simulink model "SSTI_DCDC_IET"  (R2021a)
settings: Solver=ode1  StartTime=0.0  StopTime=1.5  FixedStep=5e-6  RelTol=1e-3
values from neighbouring files (symbols this model uses):
  Pn = 1000e6    (= 1000000000)    [main_DroopCtrl_inzFDPI.m]    (also in main_PU.m)
  Sr = 10e9    (= 10000000000)    [main.m]    (also in main_DroopCtrl_inzFDPI.m)
  SYS =     [Small signal model.mat]
  Vdc1_ref = 640e3    (= 640000)    [main_DroopCtrl_inzFDPI.m]    (also in main_PU.m)
  Vdc2_ref = 500e3    (= 500000)    [main_DroopCtrl_inzFDPI.m]    (also in main_PU.m)
settings Model: Creator=Util-SHAFIQUE  LastModifiedBy=Frederic_Colas
settings SolverCC: AlgebraicLoopSolver=TrustRegion

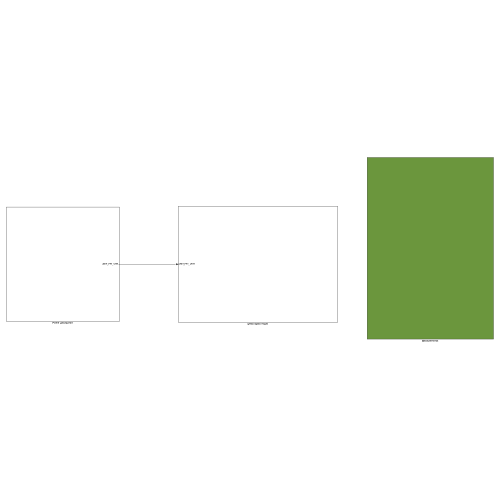
[thumbnail: Simulink's stored preview of the top-level diagram]
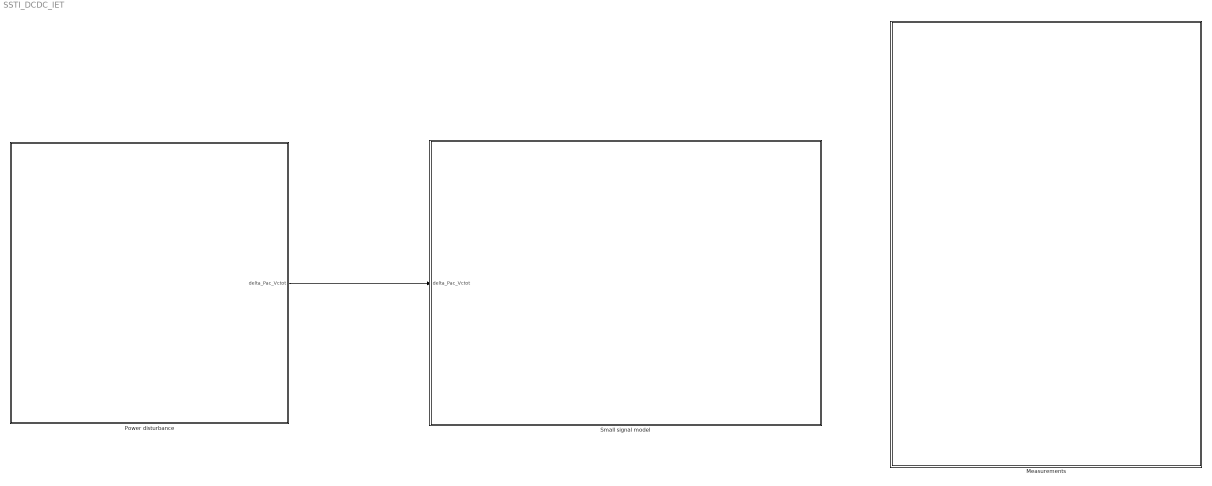
== system SSTI_DCDC_IET ==
  Measurements : Subsystem
  Power disturbance : Subsystem
  Small signal model : Subsystem
  wires:
  Power disturbance/1(delta_Pac_Vctot) -> Small signal model/1(delta_Pac_Vctot)

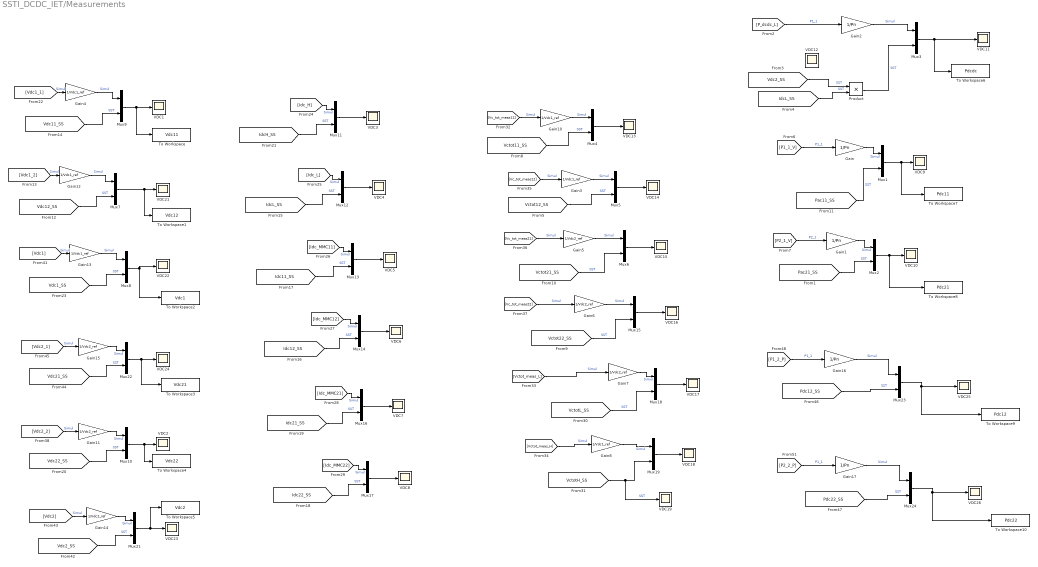
== system SSTI_DCDC_IET/Measurements ==
  Gain{,1..2,16..17} (5 alike) : Gain  Gain=1/Pn
  Gain{3..4,8,10,12..13} (6 alike) : Gain  Gain=1/Vdc1_ref
  Gain{5..7,11,14..15} (6 alike) : Gain  Gain=1/Vdc2_ref
  Mux{1..19,21..24} (23 alike) : Mux  Inputs=2
  Product : Product
  To Workspace : ToWorkspace  VariableName=Vdc11  SaveFormat=Structure With Time  SampleTime=-1
  To Workspace1 : ToWorkspace  VariableName=Vdc12  SaveFormat=Structure With Time  SampleTime=-1
  To Workspace10 : ToWorkspace  VariableName=Pdc22  SaveFormat=Structure With Time  SampleTime=-1
  To Workspace2 : ToWorkspace  VariableName=Vdc1  SaveFormat=Structure With Time  SampleTime=-1
  To Workspace3 : ToWorkspace  VariableName=Vdc21  SaveFormat=Structure With Time  SampleTime=-1
  To Workspace4 : ToWorkspace  VariableName=Vdc22  SaveFormat=Structure With Time  SampleTime=-1
  To Workspace5 : ToWorkspace  VariableName=Vdc2  SaveFormat=Structure With Time  SampleTime=-1
  To Workspace6 : ToWorkspace  VariableName=Pdcdc  SaveFormat=Structure With Time  SampleTime=-1
  To Workspace7 : ToWorkspace  VariableName=Pdc11  SaveFormat=Structure With Time  SampleTime=-1
  To Workspace8 : ToWorkspace  VariableName=Pdc21  SaveFormat=Structure With Time  SampleTime=-1
  To Workspace9 : ToWorkspace  VariableName=Pdc12  SaveFormat=Structure With Time  SampleTime=-1
  VDC{1..19,21..26} (25 alike) : Scope
  wires:
  Mux11/1 -> VDC3/1
  [Idc_L] -> Mux12/1  "Simul"
  Mux10/1 -> To Workspace4/1, VDC2/1
  [Idc_MMC12] -> Mux14/1  "Simul"
  [Vdc2_2] -> Gain11/1  "Simul"
  [Idc22_SS] -> Mux17/2  "SST"
  Mux17/1 -> VDC8/1
  Gain4/1 -> Mux9/1  "Simul"
  [Vc_tot_meas12] -> Gain3/1  "Simul"
  [Vdc1_1] -> Gain4/1  "Simul"
  Gain10/1 -> Mux4/1  "Simul"
  [Idc_H] -> Mux11/1  "Simul"
  [Vc_tot_meas21] -> Gain5/1  "Simul"
  [Vc_tot_meas11] -> Gain10/1  "Simul"
  [VctotH_SS] -> VDC19/1, Mux19/2  "SST"
  Gain3/1 -> Mux5/1  "Simul"
  Mux4/1 -> VDC13/1
  [Idc11_SS] -> Mux13/2  "SST"
  Mux12/1 -> VDC4/1
  [Idc21_SS] -> Mux16/2  "SST"
  Mux16/1 -> VDC7/1
  Mux6/1 -> VDC15/1
  Gain6/1 -> Mux15/1  "Simul"
  [Vctot22_SS] -> Mux15/2  "SST"
  Mux18/1 -> VDC17/1
  [Vctot12_SS] -> Mux5/2  "SST"
  [Vdc11_SS] -> Mux9/2  "SST"
  [IdcH_SS] -> Mux11/2  "SST"
  [Vctot11_SS] -> Mux4/2  "SST"
  Mux19/1 -> VDC18/1
  Gain5/1 -> Mux6/1  "Simul"
  [VctotL_SS] -> Mux18/2  "SST"
  Mux9/1 -> To Workspace/1, VDC1/1
  [Idc_MMC21] -> Mux16/1  "Simul"
  Gain7/1 -> Mux18/1  "Simul"
  Gain8/1 -> Mux19/1  "Simul"
  [Vctot21_SS] -> Mux6/2  "SST"
  [IdcL_SS] -> Mux12/2  "SST"
  Mux5/1 -> VDC14/1
  [Vctot_meas_L] -> Gain7/1  "Simul"
  Mux15/1 -> VDC16/1
  [Vctot_meas_H] -> Gain8/1  "Simul"
  [Vc_tot_meas22] -> Gain6/1  "Simul"
  Mux13/1 -> VDC5/1
  [Idc12_SS] -> Mux14/2  "SST"
  [Idc_MMC11] -> Mux13/1  "Simul"
  [Vdc22_SS] -> Mux10/2  "SST"
  Mux14/1 -> VDC6/1
  [Idc_MMC22] -> Mux17/1  "Simul"
  Gain11/1 -> Mux10/1  "Simul"
  [P2_1_V] -> Gain1/1  "P2_1"
  [Vdc2_SS] -> Product/1  "SST"
  Gain/1 -> Mux1/1  "Simul"
  [IdcL_SS] -> Product/2  "SST"
  [P1_1_V] -> Gain/1  "P1_1"
  Gain2/1 -> Mux3/1  "Simul"
  [Pac21_SS] -> Mux2/2  "SST"
  [Pac11_SS] -> Mux1/2  "SST"
  Gain1/1 -> Mux2/1  "Simul"
  Mux1/1 -> To Workspace7/1, VDC9/1
  Product/1 -> Mux3/2  "SST"
  [P_dcdc_L] -> Gain2/1  "P1_1"
  Mux2/1 -> To Workspace8/1, VDC10/1
  Mux3/1 -> To Workspace6/1, VDC11/1
  Mux7/1 -> To Workspace1/1, VDC21/1
  [Vdc12_SS] -> Mux7/2  "SST"
  [Vdc1_2] -> Gain12/1  "Simul"
  Gain12/1 -> Mux7/1  "Simul"
  Gain13/1 -> Mux8/1  "Simul"
  [Vdc1] -> Gain13/1  "Simul"
  [Vdc1_SS] -> Mux8/2  "SST"
  Mux8/1 -> To Workspace2/1, VDC22/1
  Gain14/1 -> Mux21/1  "Simul"
  [Vdc2_SS] -> Mux21/2  "SST"
  [Vdc2] -> Gain14/1  "Simul"
  Mux21/1 -> To Workspace5/1, VDC23/1
  Mux22/1 -> To Workspace3/1, VDC24/1
  [Vdc2_1] -> Gain15/1  "Simul"
  [Vdc21_SS] -> Mux22/2  "SST"
  Gain15/1 -> Mux22/1  "Simul"
  [P1_2_P] -> Gain16/1  "P1_1"
  Gain16/1 -> Mux23/1  "Simul"
  Mux23/1 -> To Workspace9/1, VDC25/1
  Mux24/1 -> VDC26/1, To Workspace10/1
  Gain17/1 -> Mux24/1  "Simul"
  [P2_2_P] -> Gain17/1  "P1_1"
  [Pdc12_SS] -> Mux23/2  "SST"
  [Pdc22_SS] -> Mux24/2  "SST"

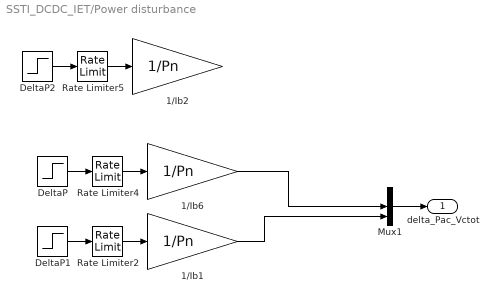
== system SSTI_DCDC_IET/Power disturbance ==
  1/Ib1 : Gain  Gain=1/Pn
  1/Ib2 : Gain  Gain=1/Pn
  1/Ib6 : Gain  Gain=1/Pn
  DeltaP : Step  Time=0.3  After=-50e6  SampleTime=0
  DeltaP1 : Step  After=50e6  SampleTime=0
  DeltaP2 : Step  Time=0.5  After=25e6  SampleTime=0
  Mux1 : Mux  Inputs=3
  Rate Limiter2 : RateLimiter  RisingSlewLimit=Sr  FallingSlewLimit=-Sr  SampleTimeMode=inherited
  Rate Limiter4 : RateLimiter  RisingSlewLimit=Sr  FallingSlewLimit=-Sr  SampleTimeMode=inherited
  Rate Limiter5 : RateLimiter  RisingSlewLimit=Sr  FallingSlewLimit=-Sr  SampleTimeMode=inherited
  delta_Pac_Vctot : Outport
  wires:
  DeltaP/1 -> Rate Limiter4/1
  DeltaP1/1 -> Rate Limiter2/1
  DeltaP2/1 -> Rate Limiter5/1
  1/Ib1/1 -> Mux1/3
  1/Ib6/1 -> Mux1/2
  Rate Limiter5/1 -> 1/Ib2/1
  Rate Limiter4/1 -> 1/Ib6/1
  Rate Limiter2/1 -> 1/Ib1/1
  Mux1/1 -> delta_Pac_Vctot/1

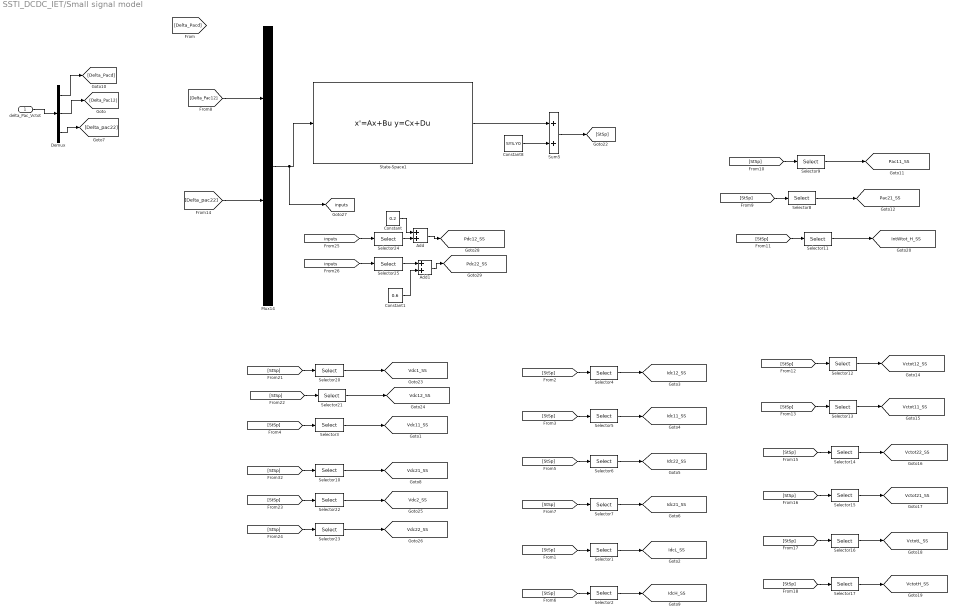
== system SSTI_DCDC_IET/Small signal model ==
  delta_Pac_Vctot : Inport
  Add : Sum
  Add1 : Sum
  Constant : Constant  Value=0.2
  Constant1 : Constant  Value=0.6
  Constant8 : Constant  Value=SYS.Y0
  Demux : Demux  Outputs=3
  Mux14 : Mux  Inputs=23
  Selector1 : Selector  InputPortWidth=46  IndexOptions=Index vector (dialog)  Indices=4  OutputSizes=1
  Selector10 : Selector  InputPortWidth=46  IndexOptions=Index vector (dialog)  Indices=43  OutputSizes=1
  Selector11 : Selector  InputPortWidth=46  IndexOptions=Index vector (dialog)  Indices=2  OutputSizes=1
  Selector12 : Selector  InputPortWidth=46  IndexOptions=Index vector (dialog)  Indices=12  OutputSizes=1
  Selector13 : Selector  InputPortWidth=46  IndexOptions=Index vector (dialog)  Indices=20  OutputSizes=1
  Selector14 : Selector  InputPortWidth=46  IndexOptions=Index vector (dialog)  Indices=32  OutputSizes=1
  Selector15 : Selector  InputPortWidth=46  IndexOptions=Index vector (dialog)  Indices=40  OutputSizes=1
  Selector16 : Selector  InputPortWidth=46  IndexOptions=Index vector (dialog)  Indices=3  OutputSizes=1
  Selector17 : Selector  InputPortWidth=46  IndexOptions=Index vector (dialog)  Indices=5  OutputSizes=1
  Selector2 : Selector  InputPortWidth=46  IndexOptions=Index vector (dialog)  Indices=6  OutputSizes=1
  Selector20 : Selector  InputPortWidth=46  IndexOptions=Index vector (dialog)  Indices=25  OutputSizes=1
  Selector21 : Selector  InputPortWidth=46  IndexOptions=Index vector (dialog)  Indices=24  OutputSizes=1
  Selector22 : Selector  InputPortWidth=46  IndexOptions=Index vector (dialog)  Indices=45  OutputSizes=1
  Selector23 : Selector  InputPortWidth=46  IndexOptions=Index vector (dialog)  Indices=44  OutputSizes=1
  Selector24 : Selector  InputPortWidth=23  IndexOptions=Index vector (dialog)  Indices=6  OutputSizes=1
  Selector25 : Selector  InputPortWidth=23  IndexOptions=Index vector (dialog)  Indices=15  OutputSizes=1
  Selector3 : Selector  InputPortWidth=46  IndexOptions=Index vector (dialog)  Indices=23  OutputSizes=1
  Selector4 : Selector  InputPortWidth=46  IndexOptions=Index vector (dialog)  Indices=14  OutputSizes=1
  Selector5 : Selector  InputPortWidth=46  IndexOptions=Index vector (dialog)  Indices=22  OutputSizes=1
  Selector6 : Selector  InputPortWidth=46  IndexOptions=Index vector (dialog)  Indices=34  OutputSizes=1
  Selector7 : Selector  InputPortWidth=46  IndexOptions=Index vector (dialog)  Indices=42  OutputSizes=1
  Selector8 : Selector  InputPortWidth=46  IndexOptions=Index vector (dialog)  Indices=46  OutputSizes=1
  Selector9 : Selector  InputPortWidth=46  IndexOptions=Index vector (dialog)  Indices=26  OutputSizes=1
  State-Space1 : StateSpace  A=SYS.A_sys  B=SYS.B_sys  C=SYS.C_sys  D=SYS.D_sys  InitialCondition=zeros(1,length(SYS.States.StrCell))
  Sum5 : Sum
  tag scope: Idc11_SS=global, Idc12_SS=global, Idc21_SS=global, Idc22_SS=global, IdcH_SS=global, IdcL_SS=global, IntWtot_H_SS=global, Pac11_SS=global, Pac21_SS=global, Pdc12_SS=global, Pdc22_SS=global, Vctot11_SS=global, Vctot12_SS=global, Vctot21_SS=global, Vctot22_SS=global, VctotH_SS=global, VctotL_SS=global, Vdc11_SS=global, Vdc12_SS=global, Vdc1_SS=global, Vdc21_SS=global, Vdc22_SS=global, Vdc2_SS=global, inputs=global
  wires:
  [StSp] -> Selector1/1
  Constant8/1 -> Sum5/2
  Selector1/1 -> [IdcL_SS]
  [StSp] -> Selector10/1
  State-Space1/1 -> Sum5/1
  Selector2/1 -> [IdcH_SS]
  Selector10/1 -> [Vdc21_SS]
  Mux14/1 -> [inputs], State-Space1/1
  Sum5/1 -> [StSp]
  [StSp] -> Selector2/1
  Selector3/1 -> [Vdc11_SS]
  [StSp] -> Selector3/1
  Demux/3 -> [Delta_pac22]
  Demux/2 -> [Delta_Pac12]
  [StSp] -> Selector5/1
  Selector5/1 -> [Idc11_SS]
  Selector4/1 -> [Idc12_SS]
  [StSp] -> Selector4/1
  [StSp] -> Selector6/1
  Selector6/1 -> [Idc22_SS]
  Selector7/1 -> [Idc21_SS]
  [StSp] -> Selector7/1
  delta_Pac_Vctot/1 -> Demux/1
  [Delta_Pac12] -> Mux14/6
  [Delta_pac22] -> Mux14/15
  Demux/1 -> [Delta_Pacd]
  [StSp] -> Selector9/1
  Selector9/1 -> [Pac11_SS]
  Selector8/1 -> [Pac21_SS]
  [StSp] -> Selector8/1
  [StSp] -> Selector15/1
  Selector15/1 -> [Vctot21_SS]
  Selector14/1 -> [Vctot22_SS]
  [StSp] -> Selector14/1
  [StSp] -> Selector12/1
  Selector12/1 -> [Vctot12_SS]
  Selector13/1 -> [Vctot11_SS]
  [StSp] -> Selector13/1
  [StSp] -> Selector17/1
  Selector17/1 -> [VctotH_SS]
  Selector16/1 -> [VctotL_SS]
  [StSp] -> Selector16/1
  Selector11/1 -> [IntWtot_H_SS]
  [StSp] -> Selector11/1
  [StSp] -> Selector20/1
  Selector20/1 -> [Vdc1_SS]
  Selector21/1 -> [Vdc12_SS]
  [StSp] -> Selector21/1
  Selector22/1 -> [Vdc2_SS]
  [StSp] -> Selector22/1
  [StSp] -> Selector23/1
  Selector23/1 -> [Vdc22_SS]
  [inputs] -> Selector25/1
  [inputs] -> Selector24/1
  Selector24/1 -> Add/2
  Selector25/1 -> Add1/1
  Add/1 -> [Pdc12_SS]
  Add1/1 -> [Pdc22_SS]
  Constant/1 -> Add/1
  Constant1/1 -> Add1/2
